simulink model "Lab6"  (R2017a)
settings: Solver=ode3  StartTime=0.0  StopTime=5  FixedStep=2e-6  RelTol=1e-5  EnableMultiTasking=on
libraries: simulink x2, commfilt2 x1, commchan3 x1, commsink2 x1, commrandsrc2 x1
settings Model: Creator=Dennis Silage  LastModifiedBy=chris
settings DataIOCC: LimitDataPoints=on  SaveFormat=Array  SignalLoggingSaveFormat=ModelDataLogs
settings OptimizationCC: ExpressionDepthLimit=2147483647  InitFltsAndDblsToZero=on  LifeSpan=inf
settings DebuggingCC: UnderspecifiedInitializationDetection=Classic  MergeDetectMultiDrivingBlocksExec=none  FcnCallInpInsideContextMsg=warning  StateNameClashWarn=warning  SFUnexpectedBacktrackingDiag=warning  SFNoUnconditionalDefaultTransitionDiag=warning  SFExecutionAtInitializationDiag=none
settings HardwareCC: ProdBitPerPointer=32  ProdBitPerSizeT=32  ProdBitPerPtrDiffT=32  ProdLargestAtomicFloat=None  ProdIntDivRoundTo=Undefined  ProdEndianess=Unspecified  ProdWordSize=32  ProdHWDeviceType=32-bit Generic
settings ModelReferenceCC: PropagateSignalLabelsOutOfModel=off
settings GRTTargetCC: TargetLangStandard=C89/C90 (ANSI)  GeneratePreprocessorConditionals=Disable all  CombineOutputUpdateFcns=off  GRTInterface=on
settings ConfigComp: CovMetricSettings=dw  CovHtmlReporting=on  CovSaveCumulativeToWorkspaceVar=on  CovSaveSingleToWorkspaceVar=on  CovExternalEMLEnable=off  CovSFcnEnable=off

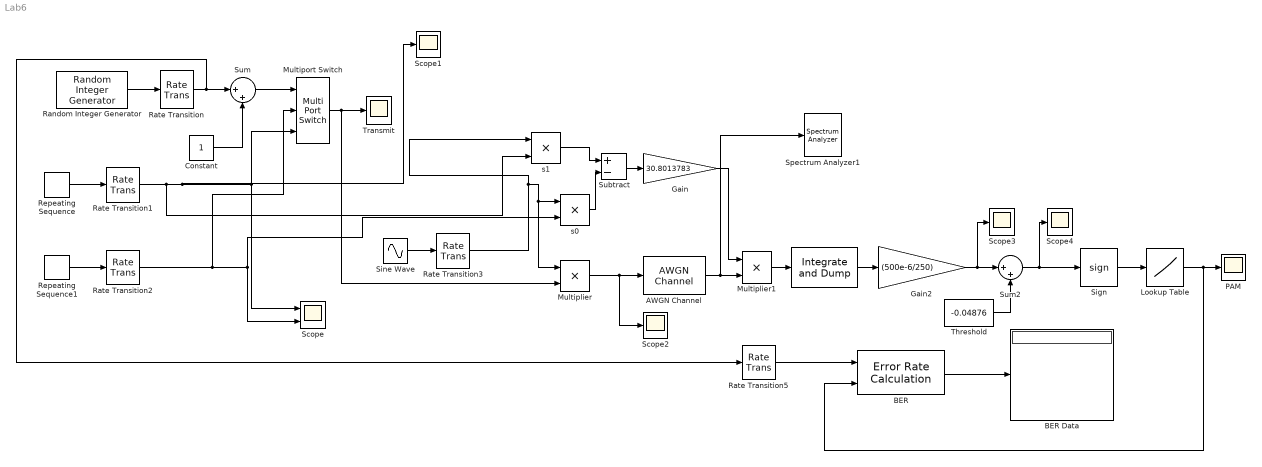
== system Lab6 ==
  " " : commfilt2/Integrate and Dump  obssamples=250  offsetsamples=0  nodump=off  roundingMode=Floor  overflowMode=on  outputDataTypeStr=Inherit: Same as accumulator  outputLastDataTypeStr=Inherit: Same as accumulator
      settings: SourceProductName=Communications System Toolbox
  AWGN Channel : commchan3/AWGN Channel  InputProcessing=Inherited (this choice will be removed - see release notes)  seed=randseed  noiseMode=Variance from mask  EbNodB=0  EsNodB=10  SNRdB=10  bitsPerSym=1  Ps=2.10809265  Tsym=500e-6  variance=0
  BER : commsink2/Error Rate Calculation  N=1  st_delay=0  cp_mode=Entire frame  subframe=[]  PMode=Port  WsName=ErrorVec  RsMode2=off  stop=off  numErr=100  maxBits=1e6
  BER Data : Display
  Constant : Constant
  Gain : Gain  Gain=30.8013783
  Gain2 : Gain  Gain=(500e-6/250)
  Lookup Table : Lookup_n-D  NumberOfTableDimensions=1  BreakpointsForDimension1=[-1, 0,1]  Table=[0,0, 1]  InternalRulePriority=Speed  RndMeth=Nearest  InputSameDT=on
  Multiplier : Product  RndMeth=Zero
  Multiplier1 : Product  RndMeth=Zero
  Multiport Switch : MultiPortSwitch  Inputs=2
  "PAM " : Scope
  Random Integer Generator : commrandsrc2/Random Integer Generator  mul=2  seed=randseed  Ts=500e-6  frameBased=off  sampPerFrame=50  orient=on  outDataType=double
  Rate Transition{,1..3} (4 alike) : RateTransition
  Rate Transition5 : RateTransition  OutPortSampleTime=500e-6
  Repeating Sequence : simulink/Sources/Repeating Sequence  rep_seq_t=[0:2e-6:125e-6 125e-6+2e-6:2e-6:500e-6]  rep_seq_y=[(.9/125e-6)*(0:2e-6:125e-6) (125e-6+2e-6:2e-6:500e-6)*0+.9]
  Repeating Sequence1 : simulink/Sources/Repeating Sequence  rep_seq_t=[0:2e-6:125e-6 125e-6+2e-6:2e-6:500e-6]  rep_seq_y=[(.45/125e-6)*(0:2e-6:125e-6) (125e-6+2e-6:2e-6:500e-6)*0+.45]
  Scope : Scope  NumInputPorts=2
  Scope{1..4} (4 alike) : Scope
  Sign : Signum
  Sine Wave : Sin  Amplitude=5  Frequency=40000*pi  SampleTime=2e-6
  Spectrum Analyzer1 : SpectrumAnalyzer
  Subtract : Sum  Inputs=+-
  Sum : Sum  Inputs=|++
  Sum2 : Sum  Inputs=|++
  Threshold : Constant  Value=-0.04876
  Transmit : Scope
  s0 : Product  RndMeth=Zero
  s1 : Product  RndMeth=Zero
  wires:
  Rate Transition/1 -> Rate Transition5/1, Sum/1
  Sum/1 -> Multiport Switch/1
  Constant/1 -> Sum/2
  Multiport Switch/1 -> Multiplier/2, Transmit/1
  BER/1 -> BER Data/1
  Sum2/1 -> Sign/1, Scope4/1
  Lookup Table/1 -> "PAM "/1, BER/2
  Random Integer Generator/1 -> Rate Transition/1
  Threshold/1 -> Sum2/2
  Sign/1 -> Lookup Table/1
  " "/1 -> Gain2/1
  Rate Transition5/1 -> BER/1
  Gain2/1 -> Sum2/1, Scope3/1
  Repeating Sequence/1 -> Rate Transition1/1
  Repeating Sequence1/1 -> Rate Transition2/1
  Sine Wave/1 -> Rate Transition3/1
  Multiplier/1 -> Scope2/1, AWGN Channel/1
  AWGN Channel/1 -> Spectrum Analyzer1/1, Multiplier1/2
  Multiplier1/1 -> " "/1
  Gain/1 -> Multiplier1/1
  Subtract/1 -> Gain/1
  s1/1 -> Subtract/1
  s0/1 -> Subtract/2
  Rate Transition1/1 -> s1/2, Scope1/1, Multiport Switch/3, Scope/1
  Rate Transition2/1 -> Multiport Switch/2, s0/2, Scope/2
  Rate Transition3/1 -> s1/1, s0/1, Multiplier/1
